simulink model "Synchronous"  (R2023b)
settings: Solver=VariableStepAuto  StartTime=0.0  StopTime=1  RelTol=1e-3
settings Model: Creator=Akaashdeep B  LastModifiedBy=Akaashdeep B

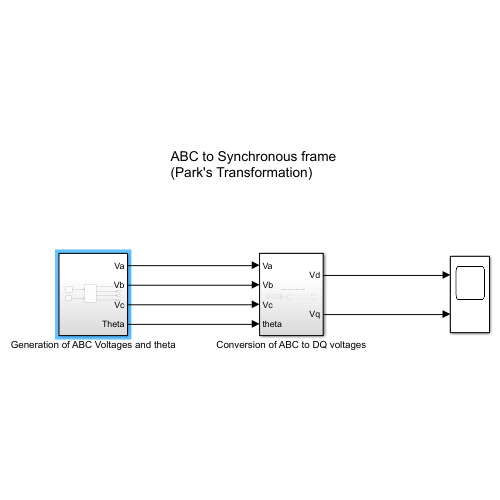
[thumbnail: Simulink's stored preview of the top-level diagram]
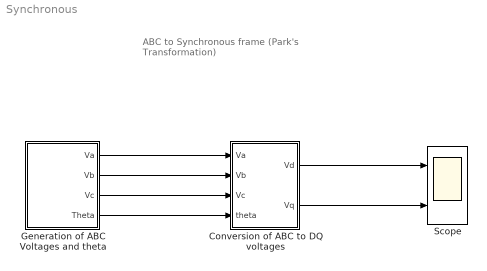
== system Synchronous ==
  note: ABC to Synchronous frame
      | (Park's Transformation)
  Conversion of ABC to DQ voltages : Subsystem
  Generation of ABC Voltages and theta : Subsystem
  Scope : Scope  NumInputPorts=2
  wires:
  Generation of ABC Voltages and theta/3(Vc) -> Conversion of ABC to DQ voltages/3(Vc)
  Generation of ABC Voltages and theta/2(Vb) -> Conversion of ABC to DQ voltages/2(Vb)
  Generation of ABC Voltages and theta/4(Theta) -> Conversion of ABC to DQ voltages/4(theta)
  Generation of ABC Voltages and theta/1(Va) -> Conversion of ABC to DQ voltages/1(Va)
  Conversion of ABC to DQ voltages/1(Vd) -> Scope/1
  Conversion of ABC to DQ voltages/2(Vq) -> Scope/2

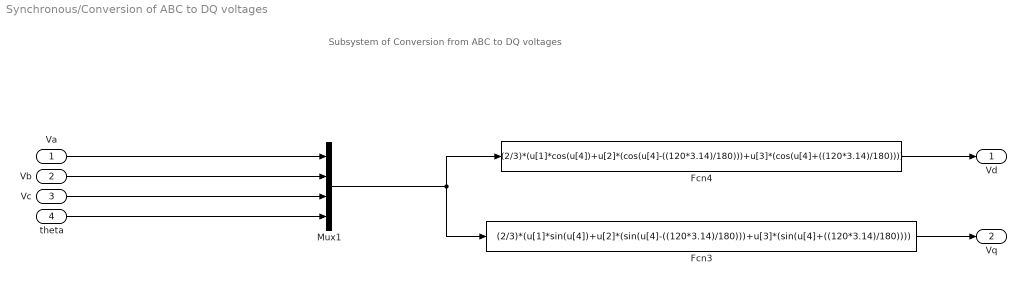
== system Synchronous/Conversion of ABC to DQ voltages ==
  note: Subsystem of Conversion from ABC to DQ voltages
  Va : Inport
  Vb : Inport  Port=2
  Vc : Inport  Port=3
  theta : Inport  Port=4
  Fcn3 : Fcn  Expr=(2/3)*(u[1]*sin(u[4])+u[2]*(sin(u[4]-((120*3.14)/180)))+u[3]*(sin(u[4]+((120*3.14)/180))))
  Fcn4 : Fcn  Expr=(2/3)*(u[1]*cos(u[4])+u[2]*(cos(u[4]-((120*3.14)/180)))+u[3]*(cos(u[4]+((120*3.14)/180))))
  Mux1 : Mux
  Vd : Outport
  Vq : Outport  Port=2
  wires:
  Va/1 -> Mux1/1
  Vb/1 -> Mux1/2
  Mux1/1 -> Fcn3/1, Fcn4/1
  theta/1 -> Mux1/4
  Fcn4/1 -> Vd/1
  Vc/1 -> Mux1/3
  Fcn3/1 -> Vq/1

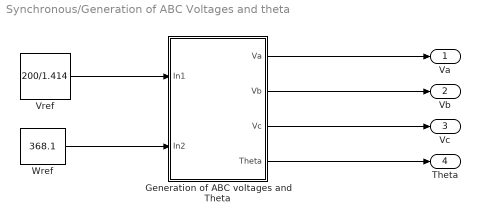
== system Synchronous/Generation of ABC Voltages and theta ==
  Generation of ABC voltages and Theta : Subsystem
  Vref : Constant  Value=200/1.414
  Wref : Constant  Value=368.1
  Va : Outport
  Vb : Outport  Port=2
  Vc : Outport  Port=3
  Theta : Outport  Port=4
  wires:
  Wref/1 -> Generation of ABC voltages and Theta/2(In2)
  Vref/1 -> Generation of ABC voltages and Theta/1(In1)
  Generation of ABC voltages and Theta/2(Vb) -> Vb/1
  Generation of ABC voltages and Theta/3(Vc) -> Vc/1
  Generation of ABC voltages and Theta/4(Theta) -> Theta/1
  Generation of ABC voltages and Theta/1(Va) -> Va/1

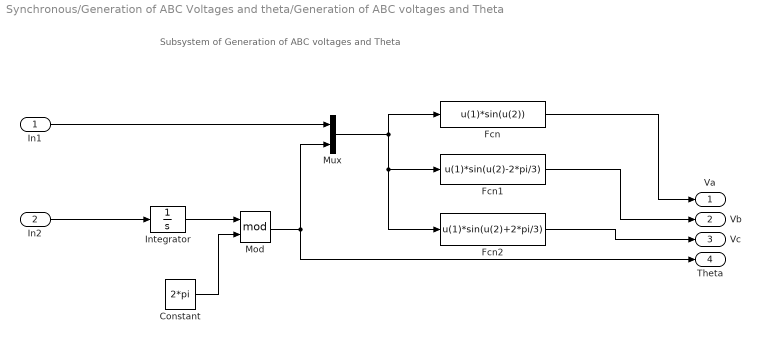
== system Synchronous/Generation of ABC Voltages and theta/Generation of ABC voltages and Theta ==
  note: Subsystem of Generation of ABC voltages and Theta
  In1 : Inport
  In2 : Inport  Port=2
  Constant : Constant  Value=2*pi
  Fcn : Fcn  Expr=u(1)*sin(u(2))
  Fcn1 : Fcn  Expr=u(1)*sin(u(2)-2*pi/3)
  Fcn2 : Fcn  Expr=u(1)*sin(u(2)+2*pi/3)
  Integrator : Integrator
  Mod : Math  Operator=mod
  Mux : Mux  Inputs=2
  Va : Outport
  Vb : Outport  Port=2
  Vc : Outport  Port=3
  Theta : Outport  Port=4
  wires:
  Mod/1 -> Theta/1, Mux/2
  Constant/1 -> Mod/2
  Mux/1 -> Fcn2/1, Fcn1/1, Fcn/1
  Fcn1/1 -> Vb/1
  Integrator/1 -> Mod/1
  Fcn/1 -> Va/1
  In1/1 -> Mux/1
  Fcn2/1 -> Vc/1
  In2/1 -> Integrator/1
